simulink model "sl_pigle_main_current"  (R2020a)
settings: Solver=VariableStepAuto  StartTime=0.0  StopTime=params.stop_time  RelTol=1e-3
PreLoadFcn:
  | load pigle_data.mat
InitFcn:
  | load pigle_data.mat
values from neighbouring files (symbols this model uses):
  params =     [pigle_data.mat]
undefined symbols (not defined in the file or in its folder): DiscIntNeverNeededParam
libraries: simulink x2, dspmtrx3 x2
settings Model: Creator=KitG  LastModifiedBy=KitG

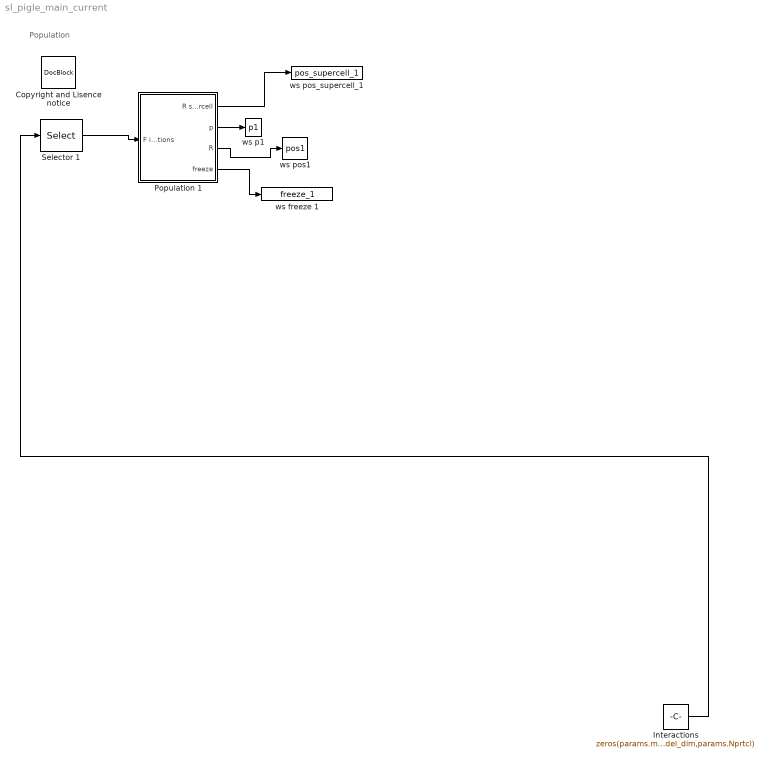
== system sl_pigle_main_current ==
  note: Population
  Copyright and Lisence notice : simulink/Model-Wide Utilities/DocBlock  DocumentType=Text
      content=|
      | % Copyright (c) 2018, Nadav Avidor.
      | % All rights reserved.
      | % This file is part of the PIGLE - Particles Interacting in Generalized Langevin Equation simulator, subject to the
      | % GNU/GPL-3.0-or-later.
  Interactions : Constant  Value=zeros(params.model_dim,params.Nprtcl)  VectorParams1D=off
  Population 1 : Subsystem
  Selector 1 : Selector  NumberOfDimensions=2  InputPortWidth=3  IndexOptions=Select all,Starting index (dialog)  Indices=,1  OutputSizes=,params.prtcl(1).Nprtcl
  ws freeze 1 : ToWorkspace  VariableName=freeze_1  SampleTime=-1
      settings: Decimation=params.decimation
  ws p1 : ToWorkspace  VariableName=p1  SampleTime=-1
      settings: Decimation=params.decimation
  ws pos1 : ToWorkspace  VariableName=pos1  SampleTime=-1
      settings: Decimation=params.decimation
  ws pos_supercell_1 : ToWorkspace  VariableName=pos_supercell_1  SampleTime=-1
      settings: Decimation=params.decimation
  wires:
  Population 1/1(R supercell) -> ws pos_supercell_1/1
  Population 1/2(p) -> ws p1/1
  Population 1/3(R) -> ws pos1/1
  Selector 1/1 -> Population 1/1(F interactions)
  Population 1/4(freeze) -> ws freeze 1/1
  Interactions/1 -> Selector 1/1

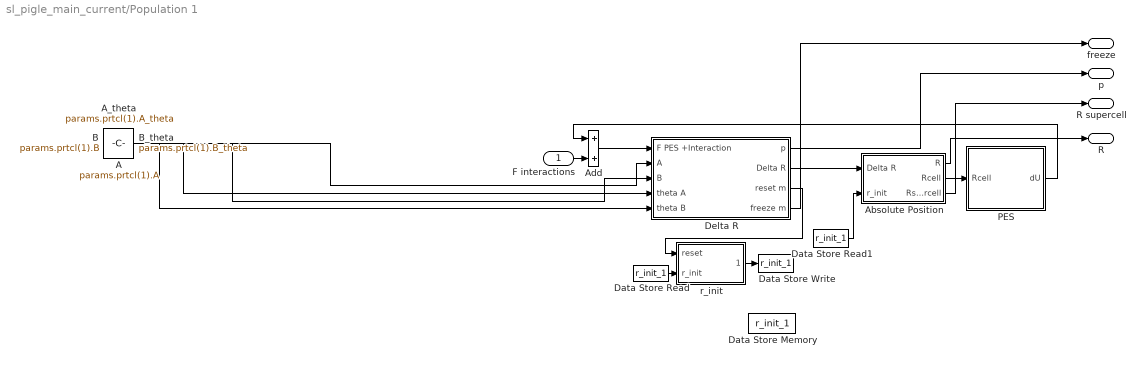
== system sl_pigle_main_current/Population 1 ==
  F interactions : Inport
  A : Constant  Value=params.prtcl(1).A  VectorParams1D=off
  A_theta : Constant  Value=params.prtcl(1).A_theta  VectorParams1D=off
  Absolute Position : Subsystem
  Add : Sum
  B : Constant  Value=params.prtcl(1).B  VectorParams1D=off
  B_theta : Constant  Value=params.prtcl(1).B_theta  VectorParams1D=off
  Data Store Memory : DataStoreMemory  DataStoreName=r_init_1  ReadBeforeWriteMsg=warning  WriteAfterWriteMsg=warning  WriteAfterReadMsg=warning  InitialValue=params.prtcl(1).r_init  VectorParams1D=off  ShowAdditionalParam=off
  Data Store Read : DataStoreRead  DataStoreName=r_init_1
  Data Store Read1 : DataStoreRead  DataStoreName=r_init_1
  Data Store Write : DataStoreWrite  DataStoreName=r_init_1
  Delta R : Subsystem
  PES : Subsystem
  r_init : Subsystem  TreatAsAtomicUnit=on
  R supercell : Outport  VectorParamsAs1DForOutWhenUnconnected=off
  p : Outport  Port=2  VectorParamsAs1DForOutWhenUnconnected=off
  R : Outport  Port=3  VectorParamsAs1DForOutWhenUnconnected=off
  freeze : Outport  Port=4  VectorParamsAs1DForOutWhenUnconnected=off
  wires:
  Delta R/4(freeze m) -> freeze/1
  r_init/1(new_r_init) -> Data Store Write/1
  Data Store Read/1 -> r_init/2(r_init)
  Data Store Read1/1 -> Absolute Position/2(r_init)
  Delta R/3(reset m) -> r_init/1(reset)
  Absolute Position/2(Rcell) -> PES/1(Rcell)
  Delta R/2(Delta R) -> Absolute Position/1(Delta R)
  Delta R/1(p) -> p/1
  PES/1(dU) -> Add/1
  Absolute Position/3(Rsupercell) -> R supercell/1
  Absolute Position/1(R) -> R/1
  F interactions/1 -> Add/2
  Add/1 -> Delta R/1(F PES +Interaction)
  A/1 -> Delta R/2(A)
  B/1 -> Delta R/3(B)
  A_theta/1 -> Delta R/4(theta A)
  B_theta/1 -> Delta R/5(theta B)

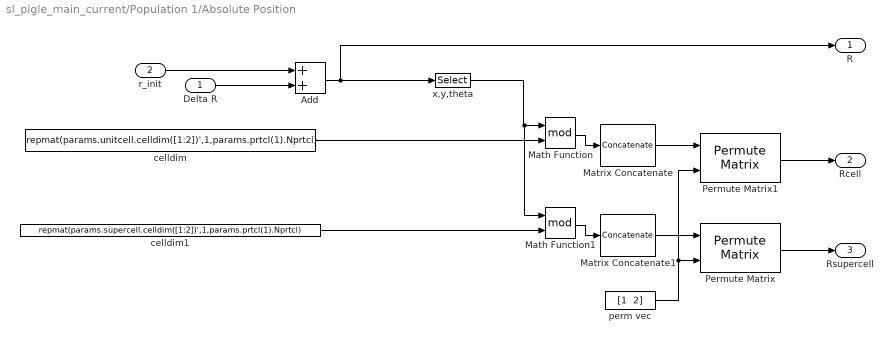
== system sl_pigle_main_current/Population 1/Absolute Position ==
  Delta R : Inport
  r_init : Inport  Port=2
  Add : Sum  Inputs=2
  Math Function : Math  Operator=mod  SignedPower=on  SaturateOnIntegerOverflow=on
  Math Function1 : Math  Operator=mod  SignedPower=on  SaturateOnIntegerOverflow=on
  Matrix Concatenate : Concatenate  NumInputs=1  Mode=Multidimensional array
  Matrix Concatenate1 : Concatenate  NumInputs=1  Mode=Multidimensional array
  Permute Matrix : dspmtrx3/Permute Matrix  mode=Rows  ZeroOneIdxMode=One-based  errmode=Generate error  checkDims=on
      settings: SourceProductBaseCode=DS
  Permute Matrix1 : dspmtrx3/Permute Matrix  mode=Rows  ZeroOneIdxMode=One-based  errmode=Generate error  checkDims=on
      settings: SourceProductBaseCode=DS
  celldim : Constant  Value=repmat(params.unitcell.celldim([1:2])',1,params.prtcl(1).Nprtcl)
  celldim1 : Constant  Value=repmat(params.supercell.celldim([1:2])',1,params.prtcl(1).Nprtcl)
  perm vec : Constant  Value="[1  2]"
  x,y,theta : Selector  NumberOfDimensions=2  InputPortWidth=3  IndexOptions=Index vector (dialog),Select all  Indices=[1:2],  OutputSizes=1,1
  R : Outport  VectorParamsAs1DForOutWhenUnconnected=off
  Rcell : Outport  Port=2  VectorParamsAs1DForOutWhenUnconnected=off
  Rsupercell : Outport  Port=3  VectorParamsAs1DForOutWhenUnconnected=off
  wires:
  Matrix Concatenate/1 -> Permute Matrix1/1
  perm vec/1 -> Permute Matrix1/2, Permute Matrix/2
  Permute Matrix1/1 -> Rcell/1
  Permute Matrix/1 -> Rsupercell/1
  Math Function/1 -> Matrix Concatenate/1
  x,y,theta/1 -> Math Function/1, Math Function1/1
  Math Function1/1 -> Matrix Concatenate1/1
  Matrix Concatenate1/1 -> Permute Matrix/1
  Add/1 -> R/1, x,y,theta/1
  celldim1/1 -> Math Function1/2
  Delta R/1 -> Add/2
  r_init/1 -> Add/1
  celldim/1 -> Math Function/2

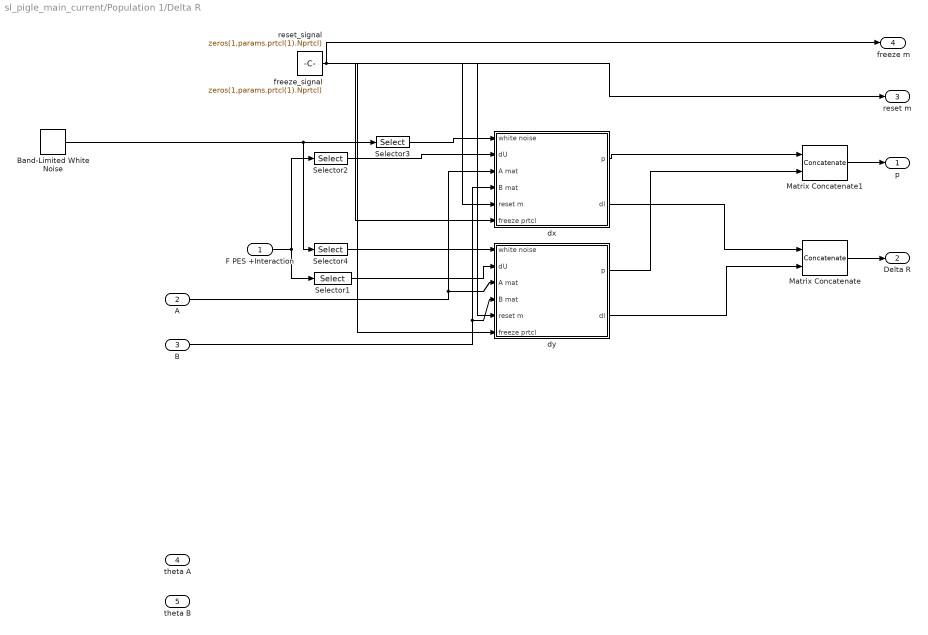
== system sl_pigle_main_current/Population 1/Delta R ==
  F PES +Interaction : Inport
  A : Inport  Port=2
  B : Inport  Port=3
  theta A : Inport  Port=4
  theta B : Inport  Port=5
  Band-Limited White Noise : simulink/Sources/Band-Limited White Noise  Cov=1  Ts=params.sample_time  seed=seed_values_1  VectorParams1D=off
  Matrix Concatenate : Concatenate  Mode=Multidimensional array
  Matrix Concatenate1 : Concatenate  Mode=Multidimensional array
  Selector1 : Selector  NumberOfDimensions=2  InputPortWidth=2  IndexOptions=Index vector (dialog),Select all  Indices=2,1  OutputSizes=1,1
  Selector2 : Selector  NumberOfDimensions=2  InputPortWidth=2  IndexOptions=Index vector (dialog),Select all  Indices=[1],1  OutputSizes=1,1
  Selector3 : Selector  NumberOfDimensions=3  InputPortWidth=2  IndexOptions=Select all,Select all,Index vector (dialog)  Indices=[1],1,1  OutputSizes=1,1,1
  Selector4 : Selector  NumberOfDimensions=3  InputPortWidth=2  IndexOptions=Select all,Select all,Index vector (dialog)  Indices=[1],1,2  OutputSizes=1,1,1
  dx : Subsystem
  dy : Subsystem
  freeze_signal : Constant  Value=zeros(1,params.prtcl(1).Nprtcl)  VectorParams1D=off
  reset_signal : Constant  Value=zeros(1,params.prtcl(1).Nprtcl)  VectorParams1D=off
  p : Outport  VectorParamsAs1DForOutWhenUnconnected=off
  Delta R : Outport  Port=2  VectorParamsAs1DForOutWhenUnconnected=off
  reset m : Outport  Port=3  VectorParamsAs1DForOutWhenUnconnected=off
  freeze m : Outport  Port=4  VectorParamsAs1DForOutWhenUnconnected=off
  wires:
  B/1 -> dy/4(B mat), dx/4(B mat)
  F PES +Interaction/1 -> Selector2/1, Selector1/1
  dy/2(dl) -> Matrix Concatenate/2
  Selector4/1 -> dy/1(white noise)
  Selector1/1 -> dy/2(dU)
  Selector2/1 -> dx/2(dU)
  Matrix Concatenate/1 -> Delta R/1
  dx/2(dl) -> Matrix Concatenate/1
  Selector3/1 -> dx/1(white noise)
  Matrix Concatenate1/1 -> p/1
  Band-Limited White Noise/1 -> Selector3/1, Selector4/1
  dy/1(p) -> Matrix Concatenate1/2
  dx/1(p) -> Matrix Concatenate1/1
  A/1 -> dy/3(A mat), dx/3(A mat)
  reset_signal/1 -> dx/5(reset m), dy/5(reset m), reset m/1
  freeze_signal/1 -> dx/6(freeze prtcl), dy/6(freeze prtcl), freeze m/1

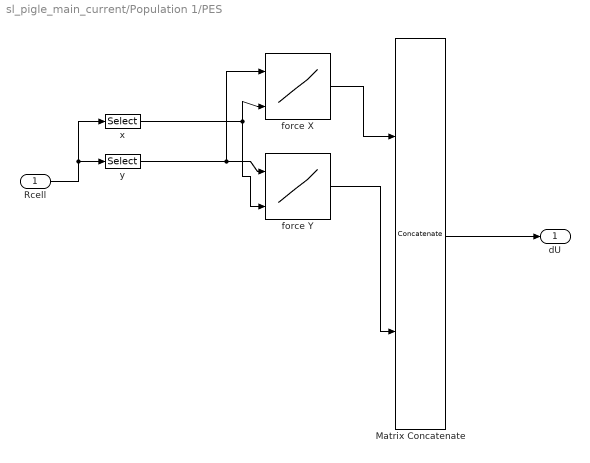
== system sl_pigle_main_current/Population 1/PES ==
  Rcell : Inport
  Matrix Concatenate : Concatenate  Mode=Multidimensional array
  force X : Lookup_n-D  BreakpointsForDimension1=params.unitcell.y  BreakpointsForDimension2=params.unitcell.x  BreakpointsForDimension3=params.unitcell.z  BreakpointsForDimension4=params.unitcell.theta  Table=params.prtcl(1).pes.fx  InternalRulePriority=Speed  RndMeth=Simplest  InputSameDT=on
  force Y : Lookup_n-D  BreakpointsForDimension1=params.unitcell.y  BreakpointsForDimension2=params.unitcell.x  BreakpointsForDimension3=params.unitcell.z  BreakpointsForDimension4=params.unitcell.theta  Table=params.prtcl(1).pes.fy  InternalRulePriority=Speed  RndMeth=Simplest  InputSameDT=on
  x : Selector  NumberOfDimensions=2  InputPortWidth=3  IndexOptions=Index vector (dialog),Select all  Indices=1,1  OutputSizes=1,1
  y : Selector  NumberOfDimensions=2  InputPortWidth=3  IndexOptions=Index vector (dialog),Select all  Indices=2,1  OutputSizes=1,1
  dU : Outport  VectorParamsAs1DForOutWhenUnconnected=off
  wires:
  Matrix Concatenate/1 -> dU/1
  Rcell/1 -> y/1, x/1
  x/1 -> force X/2, force Y/2
  force Y/1 -> Matrix Concatenate/2
  y/1 -> force X/1, force Y/1
  force X/1 -> Matrix Concatenate/1

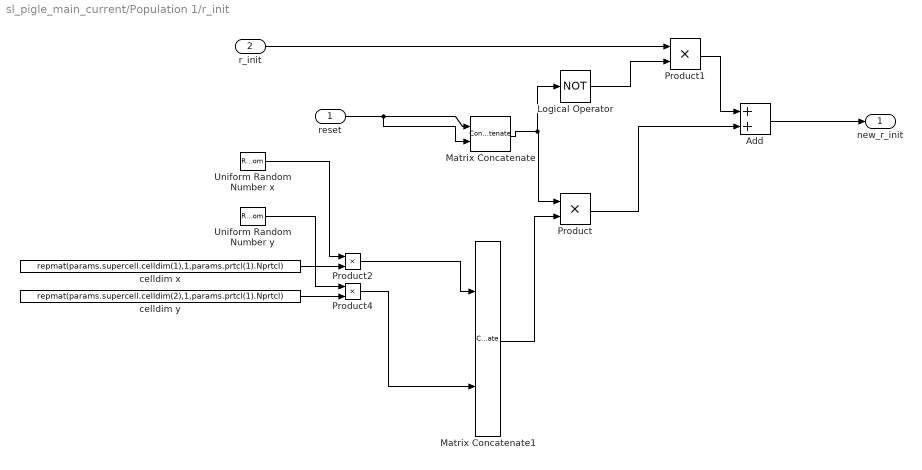
== system sl_pigle_main_current/Population 1/r_init ==
  reset : Inport
  r_init : Inport  Port=2
  Add : Sum
  Logical Operator : Logic  Operator=NOT  AllPortsSameDT=off  OutDataTypeStr=boolean
  Matrix Concatenate : Concatenate  Mode=Multidimensional array
  Matrix Concatenate1 : Concatenate  Mode=Multidimensional array
  Product{,1..2,4} (4 alike) : Product
  Uniform Random Number x : UniformRandomNumber  Minimum=0  Seed=randi(100000,1,params.prtcl(1).Nprtcl)  SampleTime=params.sample_time
  Uniform Random Number y : UniformRandomNumber  Minimum=0  Seed=randi(100000,1,params.prtcl(1).Nprtcl)  SampleTime=params.sample_time
  celldim x : Constant  Value=repmat(params.supercell.celldim(1),1,params.prtcl(1).Nprtcl)  VectorParams1D=off
  celldim y : Constant  Value=repmat(params.supercell.celldim(2),1,params.prtcl(1).Nprtcl)  VectorParams1D=off
  new_r_init : Outport  VectorParamsAs1DForOutWhenUnconnected=off
  wires:
  celldim y/1 -> Product4/2
  Uniform Random Number y/1 -> Product4/1
  r_init/1 -> Product1/1
  Product4/1 -> Matrix Concatenate1/2
  Uniform Random Number x/1 -> Product2/1
  Product2/1 -> Matrix Concatenate1/1
  celldim x/1 -> Product2/2
  Logical Operator/1 -> Product1/2
  Product1/1 -> Add/1
  reset/1 -> Matrix Concatenate/1, Matrix Concatenate/2
  Product/1 -> Add/2
  Matrix Concatenate1/1 -> Product/2
  Add/1 -> new_r_init/1
  Matrix Concatenate/1 -> Product/1, Logical Operator/1

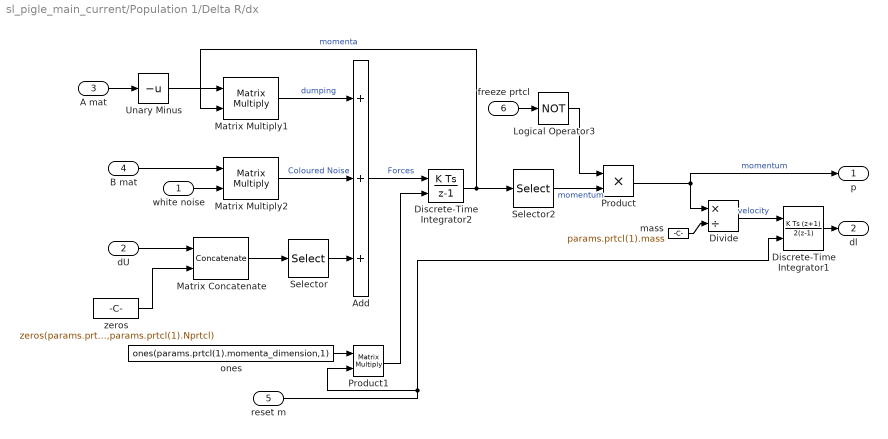
== system sl_pigle_main_current/Population 1/Delta R/dx ==
  white noise : Inport
  dU : Inport  Port=2
  A mat : Inport  Port=3
  B mat : Inport  Port=4
  reset m : Inport  Port=5
  freeze prtcl : Inport  Port=6
  Add : Sum  Inputs=+++
  Discrete-Time Integrator1 : DiscreteIntegrator  IntegratorMethod=Integration: Trapezoidal  ExternalReset=sampled level  SampleTime=-1  ICPrevOutput=DiscIntNeverNeededParam  ICPrevScaledInput=DiscIntNeverNeededParam
  Discrete-Time Integrator2 : DiscreteIntegrator  ExternalReset=sampled level  SampleTime=-1  ICPrevOutput=DiscIntNeverNeededParam  ICPrevScaledInput=DiscIntNeverNeededParam
  Divide : Product  Inputs=*/
  Logical Operator3 : Logic  Operator=NOT  AllPortsSameDT=off  OutDataTypeStr=fixdt(1,16)
  Matrix Concatenate : Concatenate  Mode=Multidimensional array
  Matrix Multiply1 : Product  Multiplication=Matrix(*)
  Matrix Multiply2 : Product  Multiplication=Matrix(*)
  Product : Product
  Product1 : Product  Multiplication=Matrix(*)
  Selector : Selector  NumberOfDimensions=2  InputPortWidth=2  IndexOptions=Index vector (dialog),Index vector (dialog)  Indices=1:params.prtcl(1).momenta_dimension,1:params.prtcl(1).Nprtcl  OutputSizes=1,1
  Selector2 : Selector  NumberOfDimensions=2  InputPortWidth=2  IndexOptions=Index vector (dialog),Select all  Indices=1,1  OutputSizes=1,1
  Unary Minus : UnaryMinus
  mass : Constant  Value=params.prtcl(1).mass
  ones : Constant  Value=ones(params.prtcl(1).momenta_dimension,1)  VectorParams1D=off
  zeros : Constant  Value=zeros(params.prtcl(1).momenta_dimension,params.prtcl(1).Nprtcl)  VectorParams1D=off
  p : Outport  VectorParamsAs1DForOutWhenUnconnected=off
  dl : Outport  Port=2  VectorParamsAs1DForOutWhenUnconnected=off
  wires:
  Logical Operator3/1 -> Product/1
  Product1/1 -> Discrete-Time Integrator2/2
  ones/1 -> Product1/1
  Selector2/1 -> Product/2  "momentum"
  Discrete-Time Integrator2/1 -> Matrix Multiply1/2, Selector2/1  "momenta"
  freeze prtcl/1 -> Logical Operator3/1
  reset m/1 -> Product1/2, Discrete-Time Integrator1/2
  dU/1 -> Matrix Concatenate/1
  Matrix Multiply2/1 -> Add/2  "Coloured Noise"
  Discrete-Time Integrator1/1 -> dl/1
  Matrix Multiply1/1 -> Add/1  "dumping"
  Product/1 -> Divide/1, p/1  "momentum"
  Add/1 -> Discrete-Time Integrator2/1  "Forces"
  B mat/1 -> Matrix Multiply2/1
  A mat/1 -> Unary Minus/1
  white noise/1 -> Matrix Multiply2/2
  Selector/1 -> Add/3
  Matrix Concatenate/1 -> Selector/1
  mass/1 -> Divide/2
  Divide/1 -> Discrete-Time Integrator1/1  "velocity"
  Unary Minus/1 -> Matrix Multiply1/1
  zeros/1 -> Matrix Concatenate/2

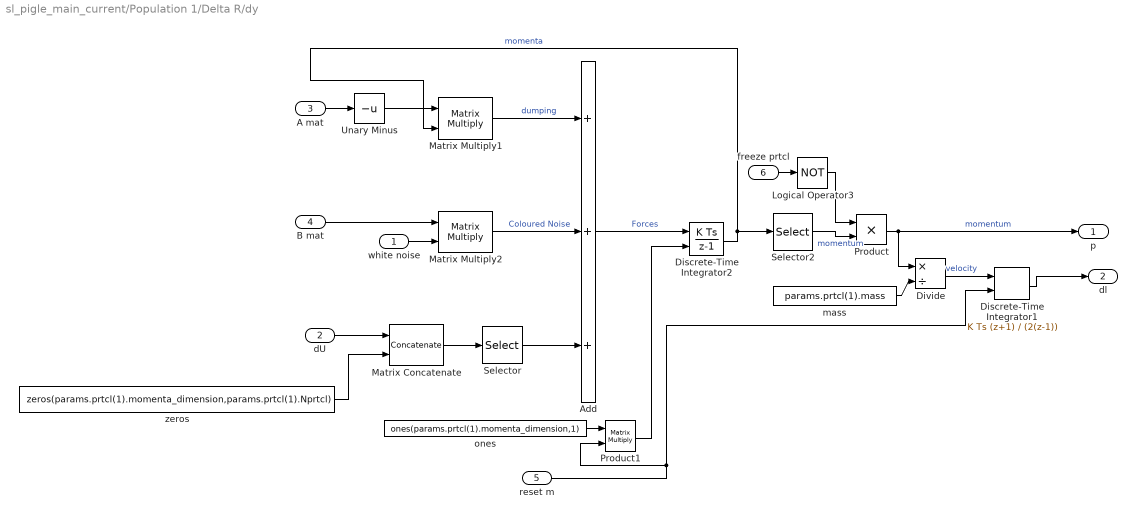
== system sl_pigle_main_current/Population 1/Delta R/dy ==
  white noise : Inport
  dU : Inport  Port=2
  A mat : Inport  Port=3
  B mat : Inport  Port=4
  reset m : Inport  Port=5
  freeze prtcl : Inport  Port=6
  Add : Sum  Inputs=+++
  Discrete-Time Integrator1 : DiscreteIntegrator  IntegratorMethod=Integration: Trapezoidal  ExternalReset=sampled level  SampleTime=-1  ICPrevOutput=DiscIntNeverNeededParam  ICPrevScaledInput=DiscIntNeverNeededParam
  Discrete-Time Integrator2 : DiscreteIntegrator  ExternalReset=sampled level  SampleTime=-1  ICPrevOutput=DiscIntNeverNeededParam  ICPrevScaledInput=DiscIntNeverNeededParam
  Divide : Product  Inputs=*/
  Logical Operator3 : Logic  Operator=NOT  AllPortsSameDT=off  OutDataTypeStr=fixdt(1,16)
  Matrix Concatenate : Concatenate  Mode=Multidimensional array
  Matrix Multiply1 : Product  Multiplication=Matrix(*)
  Matrix Multiply2 : Product  Multiplication=Matrix(*)
  Product : Product
  Product1 : Product  Multiplication=Matrix(*)
  Selector : Selector  NumberOfDimensions=2  InputPortWidth=2  IndexOptions=Index vector (dialog),Index vector (dialog)  Indices=1:params.prtcl(1).momenta_dimension,1:params.prtcl(1).Nprtcl  OutputSizes=1,1
  Selector2 : Selector  NumberOfDimensions=2  InputPortWidth=2  IndexOptions=Index vector (dialog),Select all  Indices=1,1  OutputSizes=1,1
  Unary Minus : UnaryMinus
  mass : Constant  Value=params.prtcl(1).mass
  ones : Constant  Value=ones(params.prtcl(1).momenta_dimension,1)  VectorParams1D=off
  zeros : Constant  Value=zeros(params.prtcl(1).momenta_dimension,params.prtcl(1).Nprtcl)  VectorParams1D=off
  p : Outport  VectorParamsAs1DForOutWhenUnconnected=off
  dl : Outport  Port=2  VectorParamsAs1DForOutWhenUnconnected=off
  wires:
  Logical Operator3/1 -> Product/1
  Product1/1 -> Discrete-Time Integrator2/2
  ones/1 -> Product1/1
  Selector2/1 -> Product/2  "momentum"
  freeze prtcl/1 -> Logical Operator3/1
  reset m/1 -> Product1/2, Discrete-Time Integrator1/2
  dU/1 -> Matrix Concatenate/1
  Matrix Multiply2/1 -> Add/2  "Coloured Noise"
  Discrete-Time Integrator1/1 -> dl/1
  Matrix Multiply1/1 -> Add/1  "dumping"
  Product/1 -> p/1, Divide/1  "momentum"
  Add/1 -> Discrete-Time Integrator2/1  "Forces"
  B mat/1 -> Matrix Multiply2/1
  A mat/1 -> Unary Minus/1
  white noise/1 -> Matrix Multiply2/2
  Selector/1 -> Add/3
  Discrete-Time Integrator2/1 -> Selector2/1, Matrix Multiply1/2  "momenta"
  Matrix Concatenate/1 -> Selector/1
  mass/1 -> Divide/2
  Divide/1 -> Discrete-Time Integrator1/1  "velocity"
  Unary Minus/1 -> Matrix Multiply1/1
  zeros/1 -> Matrix Concatenate/2
